simulink model "newcomplete"  (Simulink 4.00)
settings: Solver=ode45  StartTime=0.0  StopTime=300  MaxStep=0.1  RelTol=1e-3
settings Model: LastModifiedBy=Gui

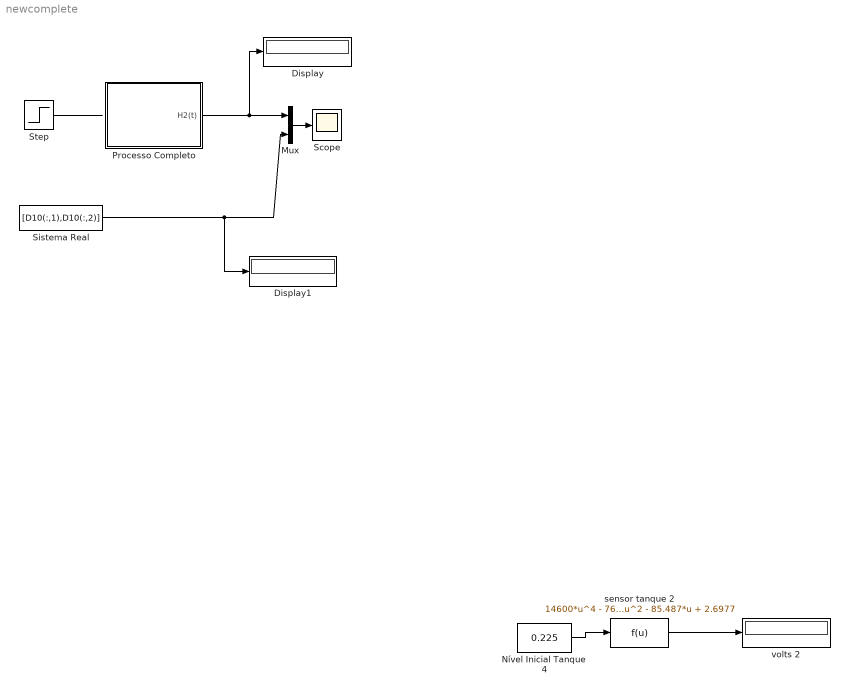
== system newcomplete ==
  Display : Display
      settings: Format=short
  Display1 : Display
      settings: Format=short
  Mux : Mux  Inputs=2
  Nível Inicial Tanque 4 : Constant  Value=0.225
  Processo Completo : Subsystem
      settings: RTWFcnNameOpts=Auto  RTWFileNameOpts=Auto
  Scope : Scope
      settings: TimeRange=auto  YMin=0  YMax=6  SaveToWorkspace=off  SaveName=ScopeData2  LimitDataPoints=on  MaxDataPoints=5000
  Sistema Real : FromWorkspace  VariableName=[D10(:,1),D10(:,2)]  SampleTime=0  OutputAfterFinalValue=Extrapolation
  Step : Step  Time=9  Before=0  After=9.998  SampleTime=0
  sensor tanque 2 : Fcn  Expr=14600*u^4 - 7625.2*u^3 + 1369.1*u^2 - 85.487*u + 2.6977
  volts 2 : Display
      settings: Format=short
  wires:
  sensor tanque 2/1 -> volts 2/1
  Nível Inicial Tanque 4/1 -> sensor tanque 2/1
  Step/1 -> ?
  Processo Completo/1("H2(t) ") -> Mux/1, Display/1
  Mux/1 -> Scope/1
  Sistema Real/1 -> Mux/2, Display1/1

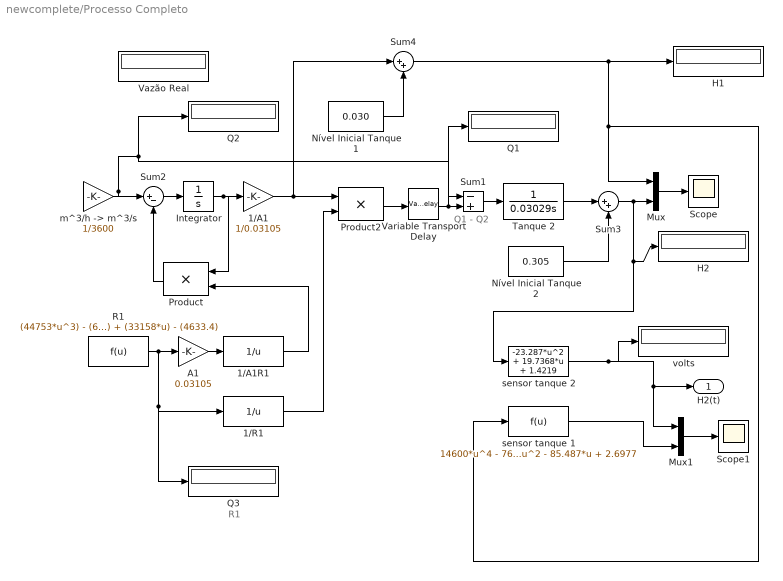
== system newcomplete/Processo Completo ==
  note: Q1 - Q2
  note: R1
  1/A1 : Gain  Gain=1/0.03105  Multiplication=Element-wise(K.*u)  SaturateOnIntegerOverflow=on
  1/A1R1 : Fcn  Expr=1/u
  1/R1 : Fcn  Expr=1/u
  A1 : Gain  Gain=0.03105  Multiplication=Element-wise(K.*u)  SaturateOnIntegerOverflow=on
  H1 : Display
      settings: Format=short
  H2 : Display
      settings: Format=short
  Integrator : Integrator  ExternalReset=none  InitialConditionSource=internal  InitialCondition=0  LimitOutput=off  UpperSaturationLimit=inf  LowerSaturationLimit=-inf  ShowSaturationPort=off  ShowStatePort=off  AbsoluteTolerance=auto
  Mux : Mux  Inputs=2
  Mux1 : Mux  Inputs=2
  Nível Inicial Tanque 1 : Constant  Value=0.030
  Nível Inicial Tanque 2 : Constant  Value=0.305
  Product : Product  Orientation=left  Inputs=2  Multiplication=Element-wise(.*)  SaturateOnIntegerOverflow=on
  Product2 : Product  Inputs=2  Multiplication=Element-wise(.*)  SaturateOnIntegerOverflow=on
  Q1 : Display
      settings: Format=short
  Q2 : Display
      settings: Format=short
  Q3 : Display
      settings: Format=short
  R1 : Fcn  Expr=(44753*u^3) - (67476*u^2) + (33158*u) - (4633.4)
  Scope : Scope
      settings: TimeRange=auto  YMin=0.161  YMax=0.1715  SaveToWorkspace=off  SaveName=ScopeData  MaxDataPoints=5000
  Scope1 : Scope
      settings: TimeRange=auto  YMin=2.4  YMax=4  SaveToWorkspace=off  MaxDataPoints=5000
  Sum1 : Sum  Inputs=-+  SaturateOnIntegerOverflow=on
  Sum2 : Sum  Inputs=|+-  SaturateOnIntegerOverflow=on
  Sum3 : Sum  Inputs=|++  SaturateOnIntegerOverflow=on
  Sum4 : Sum  Inputs=|++  SaturateOnIntegerOverflow=on
  Tanque 2 : TransferFcn  Numerator=[1]  Denominator=[0.03029 0]  AbsoluteTolerance=auto  Realization=auto
  Variable Transport Delay : VariableTransportDelay  MaximumDelay=10  InitialInput=0  MaximumPoints=1024  PadeOrder=0
  Vazão Real : Display
      settings: Format=short
  "m^3/h -> m^3/s" : Gain  Gain=1/3600  Multiplication=Element-wise(K.*u)  SaturateOnIntegerOverflow=on
  sensor tanque 1 : Fcn  Expr=14600*u^4 - 7625.2*u^3 + 1369.1*u^2 - 85.487*u + 2.6977
  "sensor tanque 2 " : Fcn  Expr=-23.287*u^2 + 19.7368*u + 1.4219
  "volts " : Display
      settings: Format=short
  "H2(t) " : Outport  Port=1
  wires:
  ? -> "m^3/h -> m^3/s"/1, Vazão Real/1, R1/1
  "m^3/h -> m^3/s"/1 -> Sum2/1, Q2/1, Sum1/1
  Integrator/1 -> Product/1, 1/A1/1
  Product/1 -> Sum2/2
  A1/1 -> 1/A1R1/1
  1/A1R1/1 -> Product/2
  R1/1 -> A1/1, 1/R1/1, Q3/1
  Sum1/1 -> Tanque 2/1
  Mux/1 -> Scope/1
  Tanque 2/1 -> Sum3/1
  Nível Inicial Tanque 2/1 -> Sum3/2
  Sum3/1 -> Mux/2, H2/1, "sensor tanque 2 "/1
  Mux1/1 -> Scope1/1
  Sum2/1 -> Integrator/1
  Product2/1 -> Variable Transport Delay/1
  Variable Transport Delay/1 -> Sum1/2, Q1/1
  "sensor tanque 2 "/1 -> "volts "/1, Mux1/1, "H2(t) "/1
  1/R1/1 -> Product2/2
  sensor tanque 1/1 -> Mux1/2
  1/A1/1 -> Sum4/1, Product2/1
  Sum4/1 -> H1/1, Mux/1, sensor tanque 1/1
  Nível Inicial Tanque 1/1 -> Sum4/2
  ? -> ?
